simulink model "scope"  (R2022a)
settings: Solver=VariableStepAuto  StartTime=0.0  StopTime=Inf  FixedStep=0.0001  RelTol=1e-3
libraries: instrumentseriallib x4, etargetslib x1, dspswit3 x1
settings Model: Creator=beatf  LastModifiedBy=beatf

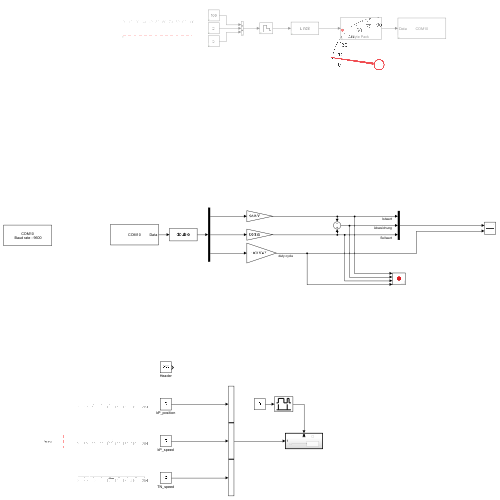
[thumbnail: Simulink's stored preview of the top-level diagram]
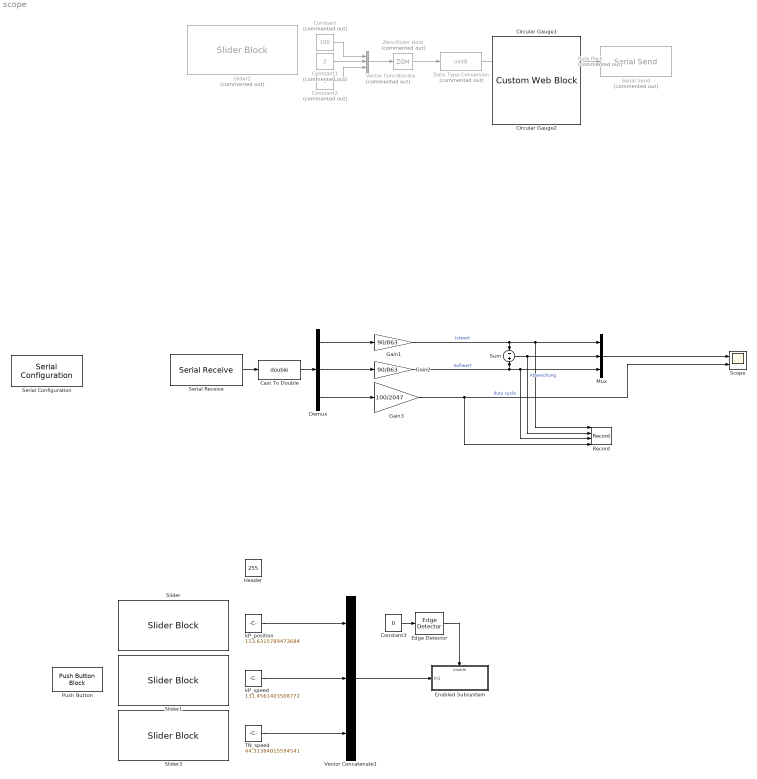
== system scope ==
  Byte Pack : etargetslib/Byte Pack  Commented=on  datatypes={'uint8'}  byteAlign=1
  Cast To Double : DataTypeConversion  OutDataTypeStr=double  SaturateOnIntegerOverflow=off  RndMeth=Floor
  Circular Gauge1 : CustomWebBlock  LabelPosition=Hide  ShowInitialText=on  Configuration="{\"components\":[{\"name\":\"CircularScaleComponent\",\"settings\":{\"bounds\":{\"max\":90,\"min\":0,\"tickInterval\":15},\"direction\":\"cw\",\"flipLimits\":0,\"innerRadius\":0.75,\"internalTickHeightScaleFactor\":1,\"labelColor\":[0,0,0],\"labelFont\":{\"font\":\"Arial\",\"fontSize\":12},\"labelRadius\":0.675074070010099,\"labelTransparency\":1,\"minorTickHeightScaleFactor\":0.2,\"needleImage\":{\"size\":[200,50],\"src\":\"data:image\\/svg+xml;base64,PD94bWwgdmVyc2lvbj0iMS4wIiBlbmNvZGluZz0idXRmLTgiPz4KPCEtLSBHZW5lcmF0b3I6IEFkb2JlIElsbHVzdHJhdG9yIDI0LjEuMiwgU1ZHIEV4cG9ydCBQbHVnLUluIC4gU1ZHIFZlcnNpb246IDYuMDAgQnVpbGQgMCkgIC0tPgo8c3ZnIHZlcnNpb249IjEuMSIgaWQ9IkxheWVyXzEiIHhtbG5zPSJodHRwOi8vd3d3LnczLm9yZy8yMDAwL3N2ZyIgeG1sbnM6eGxpbms9Imh0dHA6Ly93d3cudzMub3JnLzE5OTkveGxpbmsiIHg9IjBweCIgeT0iMHB4IgoJIHZpZXdCb3g9IjAgMCAyMDAgNTAiIHN0eWxlPSJlbmFibGUtYmFja2dyb3VuZDpuZXcgMCAwIDIwMCA1MDsiIHhtbDpzcGFjZT0icHJlc2VydmUiPgo8c3R5bGUgdHlwZT0idGV4dC9jc3MiPgoJLnN0MHtmaWxsOiNFQzIxMjc7fQo8L3N0eWxlPgo8cGF0aCBjbGFzcz0ic3QwIiBkPSJNMTYyLjgsMTMuN0MxNjksNC40LDE4MS43LDEuOSwxOTEsOC4xczExLjgsMTguOSw1LjYsMjguMnMtMTguOSwxMS44LTI4LjIsNS42bDAsMAoJQzE1OS4xLDM1LjYsMTU2LjYsMjMsMTYyLjgsMTMuN0wxNjIuOCwxMy43eiBNMTY1LjgsMTUuOGMtNS4xLDcuNi0zLjEsMTcuOSw0LjYsMjNjNy42LDUuMSwxNy45LDMuMSwyMy00LjYKCWM1LjEtNy42LDMuMS0xNy45LTQuNi0yM2wwLDBDMTgxLjIsNi4yLDE3MC45LDguMiwxNjUuOCwxNS44eiIvPgo8cGF0aCBjbGFzcz0ic3QwIiBkPSJNMC40LDI1Ljl2LTMuM2wxNTktMi41Yy0wLjcsMi42LTAuNyw1LjIsMCw3LjhMMC40LDI1Ljl6Ii8+CjxjaXJjbGUgY2xhc3M9InN0MCIgY3g9IjE3OS42IiBjeT0iMjQiIHI9IjAuNyIvPgo8L3N2Zz4K\"},\"needleOffset\":[0.18464878250906522,0],\"needleOrientation\":-45,\"needleRotation\":180,\"needleSize\":{\"height\":0.11741692305346914,\"width\":0.46108337545091255},\"outerRadius\":0.8,\"position\":[-0.1,-0.1,2,2],\"referencePoint\":\"auto\",\"scaleAngle\":90,\"scaleAngleOffset\":180,\"scaleColors\":[],\"scaleColorsSize\":0.2,\"scaleDirection\":\"CW\",\"scalePosition\":[0,0,1,1],\"showLabels\":1,\"showMinorTicks\":1,\"showSpanLine\":1,\"showTicks\":1,\"tickColor\":[0,0,0],\"tickTransparency\":1,\"valueBarColor\":[0,114,189],\"valueBarPosition\":[0,0,1,1],\"valueBarSize\":0.2,\"valueBarTransparency\":0}},{\"name\":\"BackgroundImageComponent\",\"settings\":{\"image\":{\"size\":[0,0],\"src\":\"default\"},\"position\":[0,0,1,1],\"scaleMode\":\"0\"}},{\"name\":\"ForegroundImageComponent\",\"settings\":{\"image\":{\"size\":[0,0],\"src\":\"default\",\"srcOrientation\":[]},\"isForeground\":1,\"position\":[0,0,1,1],\"scaleMode\":\"0\"}}],\"settings\":{\"BindingType\":\"signal\",\"aspectRatio\":1.032258064516129,\"backgroundColor\":[0,0,0,\"1\"],\"backgroundOffset\":0.14,\"backgroundOpacity\":1,\"direction\":\"cw\",\"fixedAspectRatio\":\"on\",\"flipLimits\":0,\"orientation\":\"horizontal\",\"showBackgroundColor\":false,\"value\":0},\"type\":\"CircularGauge\"}"
  Circular Gauge2 : CustomWebBlock  LabelPosition=Hide  ShowInitialText=on  Configuration="{\"components\":[{\"name\":\"CircularScaleComponent\",\"settings\":{\"bounds\":{\"max\":90,\"min\":0,\"tickInterval\":15},\"direction\":\"cw\",\"flipLimits\":0,\"innerRadius\":0.75,\"internalTickHeightScaleFactor\":1,\"labelColor\":[0,0,0],\"labelFont\":{\"font\":\"Arial\",\"fontSize\":12},\"labelRadius\":0.675074070010099,\"labelTransparency\":1,\"minorTickHeightScaleFactor\":0.2,\"needleImage\":{\"size\":[200,50],\"src\":\"data:image\\/png;base64,iVBORw0KGgoAAAANSUhEUgAAAMgAAAAyCAYAAAAZUZThAAAACXBIWXMAAAsTAAALEwEAmpwYAAACuklEQVR4nO3bzWoTYRSH8f+YhLZDY8mmkEUbCRTaO4gVqqS4lC6UFtRNoRtvoa69BndmY4sVd+4sirYqwRtooTAwtTrQTdDpZ5IaF4n1o\\/rShiMO8vyWgZOcRR6SGd7xWq2WAPzeuX+9AJBkBAI4EAjgQCCAA4EADgQCOBAI4EAggAOBAA4EAjgQCOBAIIADgQAOBAI4EAjgQCCAQ9rkXTzvxEvFQr4saUZSWdJw5+VNSS8kPQ7C6PmJIR7eQsJ4Jk8U\\/hBIsZAflXR\\/rN64cn13XxP7hxpuHkmSNtMprfT1aKnf10Ym\\/VLSnSCM1o+HCQQJYxpIsZC\\/3NtqPZ2vfc7ejPf++P\\/tSNKjrK97ufPxgeddC8LolSQCQeKYBVIs5EczrVb1wXZt4NLB4anG3vb2aHYw96nheaUgjNYJBEljcpFeLOQ9SZW7tfjUcUjS+MGh5mvxgKRK5z2ARLG6izU50miWbsW7Zx68He9qpNEsSZo02gUwYxXI9MzOnlJdDKYkzezsSdK00S6AGatAyhP7p\\/9r9avObNloF8CMVSBDhc6t3G50bgMPGe0CmLEKpPufD0lNoyUAa1aBfAzT3VyBtH1oz24Z7QKYsQrk3UpfT9fDq+3ZN0a7AGasAllY6vfVzVXIkaSlfl+SHhrtApixCuTZRiZdXcz6Zx5czPrayKSrkpaNdgHMmB81qWzXBsbPftTkYhBGaxw1QdKYPQ8ShNF6w\\/Om5gZz8ULWl+ur\\/kXSQtbX3GAubnjeVBBGa1Z7AJb+1nH3yli9Ufp23P1Cs6m6PG2lU3r9\\/bh7VdIsx92RZOaBSMeHF69KuqH2GashSXVJ7yWtSnoiaTkIo58\\/nECQMDaBAP8pnkkHHAgEcCAQwIFAAAcCARwIBHAgEMCBQAAHAgEcCARwIBDAgUAABwIBHAgEcPgKyyrQblWfvigAAAAASUVORK5CYII=\"},\"needleOffset\":[0.315,0],\"needleOrientation\":-45,\"needleRotation\":180,\"needleSize\":{\"height\":0.07,\"width\":0.3},\"outerRadius\":0.8,\"position\":[-0.1,-0.1,2,2],\"referencePoint\":\"auto\",\"scaleAngle\":90,\"scaleAngleOffset\":180,\"scaleColors\":[],\"scaleColorsSize\":0.2,\"scaleDirection\":\"CW\",\"scalePosition\":[0,0,1,1],\"showLabels\":false,\"showMinorTicks\":1,\"showSpanLine\":false,\"showTicks\":false,\"tickColor\":[0,0,0],\"tickTransparency\":1,\"valueBarColor\":[0,114,189],\"valueBarPosition\":[0,0,1,1],\"valueBarSize\":0.2,\"valueBarTransparency\":0}},{\"name\":\"BackgroundImageComponent\",\"settings\":{\"image\":{\"size\":[0,0],\"src\":\"default\"},\"position\":[0,0,1,1],\"scaleMode\":\"0\"}},{\"name\":\"ForegroundImageComponent\",\"settings\":{\"image\":{\"size\":[0,0],\"src\":\"default\",\"srcOrientation\":[]},\"isForeground\":1,\"position\":[0,0,1,1],\"scaleMode\":\"0\"}}],\"settings\":{\"BindingType\":\"signal\",\"aspectRatio\":1.032258064516129,\"backgroundColor\":[0,0,0,\"1\"],\"backgroundOffset\":0.14,\"backgroundOpacity\":1,\"direction\":\"cw\",\"fixedAspectRatio\":\"on\",\"flipLimits\":0,\"orientation\":\"horizontal\",\"showBackgroundColor\":false,\"value\":0},\"type\":\"CircularGauge\"}"
  Constant : Constant  Commented=on  Value=100
  Constant1 : Constant  Commented=on  Value=2
  Constant2 : Constant  Commented=on  Value=3
  Constant3 : Constant  Value=0
  Data Type Conversion : DataTypeConversion  Commented=on  OutDataTypeStr=uint8  SaturateOnIntegerOverflow=off  RndMeth=Floor
  Demux : Demux  Outputs=3
  Edge Detector : dspswit3/Edge Detector  InputProcessing=Columns as channels (frame based)
      settings: SourceProductBaseCode=DS
  Enabled Subsystem : Subsystem  TreatAsAtomicUnit=on
  Gain1 : Gain  Gain=90/863
  Gain2 : Gain  Gain=90/863
  Gain3 : Gain  Gain=100/2047
  Header : Constant  Value=255  OutDataTypeStr=uint8
  Mux : Mux  Inputs=3
  Push Button : PushButtonBlock  ButtonText=Send  OffValue=0.000000
  Record : Record  FileSettingsInternal="{\"entries\":[{\"content\":{\"excelSettings\":{\"content\":{},\"type\":\"Streamout.ExcelSettings\"}},\"type\":\"Streamout.FileSettingStorage\",\"uuid\":\"773e9e15-1439-4f98-85d8-032cda1a1bf1\"}],\"packageUris\":[\"http://schema.mathworks.com/mf0/streamout_blocks/R2020a\"],\"version\":\"1.0\"}"  SignalsInternal="{\"entries\":[{\"content\":{\"signals\":[{\"content\":{\"blockPath\":[\"scope_fef9decd5c/Record\"],\"channel\":[],\"dimensions\":[1,1],\"domain\":\"scope_fef9decd5c/Record\",\"lineColor\":\"#a2142f\",\"plots\":[1],\"port\":1,\"sid\":[\"\"],\"signalID\":703,\"signalName\":\"Istwert\"},\"type\":\"RecordBlkView.Signal\",\"uuid\":\"5c3736ea-e8b3-408c-8d24-98182dbffe17\"},{\"content\":{\"blockPath\":[\"scope_fef9decd5c/Record\"],\"channel\":[],\"dimensions\":[1,1],\"domain\":\"scope_fef9decd5c/Record\",\"lineColor\":\"#139fff\",\"plots\":[1],\"port\":2,\"sid\":[\"\"],\"signalID\":707,\"signalName\":\"Abweichung\"},\"type\":\"RecordBlkView.Signal\",\"uuid\":\"64b213d3-799d-4729-b2cd-248f93a9f961\"},{\"content\":{\"blockPath\":[\"scope_fef9decd5c/Record\"],\"channel\":[],\"dimensions\":[1,1],\"domain\":\"scope_fef9decd5c/Record\",\"lineColor\":\"#ff6929\",\"plots\":[1],\"port\":3,\"sid\":[\"\"],\"signalID\":711,\"signalName\":\"Sollwert\"},\"type\":\"RecordBlkView.Signal\",\"uuid\":\"d6159f83-069e-4e2a-938d-c786a59cdc26\"},{\"content\":{\"blockPath\":[\"scope_fef9decd5c/Record\"],\"channel\":[],\"dimensions\":[1,1],\"domain\":\"scope_fef9decd5c/Record\",\"lineColor\":\"#b746ff\",\"plots\":[1],\"port\":4,\"sid\":[\"\"],\"signalID\":715,\"signalName\":\"duty cycle\"},\"type\":\"RecordBlkView.Signal\",\"uuid\":\"0e45bb36-03b6-4bca-809d-3a40864760f6\"}]},\"type\":\"RecordBlkView.InputSignals\",\"uuid\":\"a81651cf-620c-4893-944e-ea50361a1552\"}],\"packageUris\":[\"http://schema.mathworks.com/mf0/streamout_blocks/R2020a\"],\"version\":\"1.0\"}"  VisualizationBindings="{\"sparklinesplugin\":{\"info\":[{\"bindingParametersList\":[],\"subplotID\":1}]}}"
  Scope : Scope  NumInputPorts=2
  Serial Configuration : instrumentseriallib/Serial Configuration  Priority=-200000  PortSel=COM10  Port=COM10  ComPort=COM10  BaudRate=9600  DataBits=8  Parity=none  StopBits=1  ByteOrder=little-endian  FlowControl=none  Timeout=10  SimulateUsing=Interpreted execution  BlockInModel=on  aMode=1
      settings: SourceProductBaseCode=OT,IC,MT
  Serial Receive : instrumentseriallib/Serial Receive  Priority=1  PortSel=COM10  Port=COM10  ComPort=COM10  DataType=uint16  SaveDataType=uint8  ToggleHeader=on  Header=[255 0 100]  ToggleTerminator=off  Terminator=<none>  CustomTerminator=[]  InputFormat=Column major  ToggleDataSize=on  DataSize=[1 3]  EnableBlockingMode=on  ActionDataUnavailable=Output last received value  ActionWhenDataUnavailable=Output last received value  CustomValue=0  SampleTime=0.01  SimulateUsing=Interpreted execution  BlockInModel=on  aMode=1
      settings: SourceProductBaseCode=OT,IC,MT
  Serial Send : instrumentseriallib/Serial Send  Priority=1  Commented=on  PortSel=COM10  Port=COM10  ComPort=COM10  Header=[255]  Terminator=<none>  CustomTerminator=[]  EnableBlockingMode=on  SimulateUsing=Interpreted execution  BlockInModel=on  aMode=1
      settings: SourceProductBaseCode=OT,IC,MT
  Slider : SliderBlock  ScaleMax=254
  Slider1 : SliderBlock  ScaleMax=254
  Slider2 : SliderBlock  Commented=on
  Slider3 : SliderBlock  ScaleMax=254
  Sum : Sum  Inputs=-|+  AccumDataTypeStr=int32  OutDataTypeStr=Inherit: Same as first input
  TN_speed : Constant  Value=44.31384015594541  OutDataTypeStr=uint8
  Vector Concatenate : Concatenate  Commented=on  NumInputs=3
  Vector Concatenate1 : Concatenate  NumInputs=3
  Zero-Order Hold : ZeroOrderHold  Commented=on  SampleTime=2
  kP_position : Constant  Value=113.6315789473684  OutDataTypeStr=uint8
  kP_speed : Constant  Value=131.4561403508772  OutDataTypeStr=uint8
  wires:
  Gain1/1 -> Record/1, Mux/1, Sum/1  "Istwert"
  Sum/1 -> Mux/2, Record/2  "Abweichung"
  Gain3/1 -> Scope/2, Record/4  "duty cycle"
  Serial Receive/1 -> Cast To Double/1
  Demux/3 -> Gain3/1
  Demux/1 -> Gain1/1
  Demux/2 -> Gain2/1
  Gain2/1 -> Mux/3, Record/3, Sum/2  "Sollwert"
  Constant/1 -> Vector Concatenate/1
  Constant1/1 -> Vector Concatenate/2
  Constant2/1 -> Vector Concatenate/3
  Vector Concatenate/1 -> Zero-Order Hold/1
  Data Type Conversion/1 -> Byte Pack/1
  Byte Pack/1 -> Serial Send/1
  Zero-Order Hold/1 -> Data Type Conversion/1
  kP_position/1 -> Vector Concatenate1/1
  kP_speed/1 -> Vector Concatenate1/2
  TN_speed/1 -> Vector Concatenate1/3
  Constant3/1 -> Edge Detector/1
  Edge Detector/1 -> Enabled Subsystem/Enable
  Vector Concatenate1/1 -> Enabled Subsystem/1(In1)
  Mux/1 -> Scope/1
  Cast To Double/1 -> Demux/1

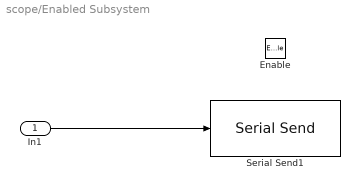
== system scope/Enabled Subsystem ==
  In1 : Inport
  Enable : EnablePort
  Serial Send1 : instrumentseriallib/Serial Send  Priority=1  PortSel=COM10  Port=COM10  ComPort=COM10  Header=[]  Terminator=<none>  CustomTerminator=[]  EnableBlockingMode=off  SimulateUsing=Interpreted execution  BlockInModel=on  aMode=1
      settings: SourceProductBaseCode=OT,IC,MT
  wires:
  In1/1 -> Serial Send1/1
